simulink model "ADPSEMREMKNNash2015b"  (R2016a)
settings: Solver=ode1  StartTime=0.0  StopTime=40  FixedStep=1/1000  RelTol=1e-3  AbsTol=1e-3
PostLoadFcn:
  | f_Simulink_figureplace
InitFcn:
  | ADPSEMREMKNNash_PreSim
values from neighbouring files (symbols this model uses):
  beta1 = 0.3    [ADPSEMREMKNNash_PreSim.m]
  beta2 = 0.3    [ADPSEMREMKNNash_PreSim.m]
  beta3 = 0.3    [ADPSEMREMKNNash_PreSim.m]
  beta4 = 0.2    [ADPSEMREMKNNash_PreSim.m]
  beta5 = 0.1    [ADPSEMREMKNNash_PreSim.m]
  etaa11 = 1    [ADPSEMREMKNNash_PreSim.m]
  etaa12 = 0.5    [ADPSEMREMKNNash_PreSim.m]
  etaa13 = 1    [ADPSEMREMKNNash_PreSim.m]
  etaa14 = 0.5    [ADPSEMREMKNNash_PreSim.m]
  etaa15 = 1    [ADPSEMREMKNNash_PreSim.m]
  etaa21 = 2    [ADPSEMREMKNNash_PreSim.m]
  etaa22 = 1.5    [ADPSEMREMKNNash_PreSim.m]
  etaa23 = 2    [ADPSEMREMKNNash_PreSim.m]
  etaa24 = 1    [ADPSEMREMKNNash_PreSim.m]
  etaa25 = 1    [ADPSEMREMKNNash_PreSim.m]
  etac11 = 0.05    [ADPSEMREMKNNash_PreSim.m]
  etac12 = 0.001    [ADPSEMREMKNNash_PreSim.m]
  etac13 = 0.001    [ADPSEMREMKNNash_PreSim.m]
  etac14 = 0.001    [ADPSEMREMKNNash_PreSim.m]
  etac15 = 0.001    [ADPSEMREMKNNash_PreSim.m]
  etac21 = 5    [ADPSEMREMKNNash_PreSim.m]
  etac22 = 5    [ADPSEMREMKNNash_PreSim.m]
  etac23 = 5    [ADPSEMREMKNNash_PreSim.m]
  etac24 = 5    [ADPSEMREMKNNash_PreSim.m]
  etac25 = 5    [ADPSEMREMKNNash_PreSim.m]
  Gamma01 = 20*eye(L1)    [ADPSEMREMKNNash_PreSim.m]
  Gamma02 = 30*eye(L2)    [ADPSEMREMKNNash_PreSim.m]
  Gamma03 = 30*eye(L3)    [ADPSEMREMKNNash_PreSim.m]
  Gamma04 = 50*eye(L4)    [ADPSEMREMKNNash_PreSim.m]
  Gamma05 = 100*eye(L5)    [ADPSEMREMKNNash_PreSim.m]
  L5 = size(sig_p,1)    [ADPSEMREMKNN_Basis5.m]
  MovePoints = 1    [ADPSEMREMKNNash_PreSim.m]
  n = 3    [ADPSEMREMKNNash_PreSim.m]
  Q1 = [10 0 0; 0 10 0; 0 0 10]    [ADPSEMREMKNNash_PreSim.m]
  Q2 = [10 0 0; 0 10 0; 0 0 10]    [ADPSEMREMKNNash_PreSim.m]
  Q3 = [10 0 0; 0 10 0; 0 0 10]    [ADPSEMREMKNNash_PreSim.m]
  Q4 = [10 0 0; 0 10 0; 0 0 10]    [ADPSEMREMKNNash_PreSim.m]
  Q5 = [10 0 0; 0 10 0; 0 0 10]    [ADPSEMREMKNNash_PreSim.m]
  R1 = 1    [ADPSEMREMKNNash_PreSim.m]
  R2 = 1    [ADPSEMREMKNNash_PreSim.m]
  R3 = 1    [ADPSEMREMKNNash_PreSim.m]
  R4 = 1    [ADPSEMREMKNNash_PreSim.m]
  R5 = 1    [ADPSEMREMKNNash_PreSim.m]
  s1 = 0.25    [ADPSEMREMKNNash_PreSim.m]
  s2 = 0.25    [ADPSEMREMKNNash_PreSim.m]
  s3 = 0.25    [ADPSEMREMKNNash_PreSim.m]
  s4 = 0.25    [ADPSEMREMKNNash_PreSim.m]
  s5 = 0.25    [ADPSEMREMKNNash_PreSim.m]
  v1 = 1    [ADPSEMREMKNNash_PreSim.m]
  v2 = 1    [ADPSEMREMKNNash_PreSim.m]
  v3 = 1    [ADPSEMREMKNNash_PreSim.m]
  v4 = 1    [ADPSEMREMKNNash_PreSim.m]
  v5 = 1    [ADPSEMREMKNNash_PreSim.m]
  WaH01 = 2*ones(L1,1)    [ADPSEMREMKNNash_PreSim.m]
  WaH02 = 2*ones(L2,1)    [ADPSEMREMKNNash_PreSim.m]
  WaH03 = 2*ones(L3,1)    [ADPSEMREMKNNash_PreSim.m]
  WaH04 = 1*ones(L4,1)    [ADPSEMREMKNNash_PreSim.m]
  WaH05 = 1*ones(L5,1)    [ADPSEMREMKNNash_PreSim.m]
  WcH01 = 5*ones(L1,1)    [ADPSEMREMKNNash_PreSim.m]
  WcH02 = 2*ones(L2,1)    [ADPSEMREMKNNash_PreSim.m]
  WcH03 = 2*ones(L3,1)    [ADPSEMREMKNNash_PreSim.m]
  WcH04 = 5*ones(L4,1)    [ADPSEMREMKNNash_PreSim.m]
  WcH05 = 2*ones(L5,1)    [ADPSEMREMKNNash_PreSim.m]
  x01 = [0; 0; 0]    [ADPSEMREMKNNash_PreSim.m]
  x02 = [0; 0; 0]    [ADPSEMREMKNNash_PreSim.m]
  x03 = [0; 0; 0]    [ADPSEMREMKNNash_PreSim.m]
  x04 = 0*[0.5; -0.5; 0]    [ADPSEMREMKNNash_PreSim.m]
  x05 = 0*[-0.5; -0.5; 0]    [ADPSEMREMKNNash_PreSim.m]
  xd21 = [0.5;-0.5;0]    [ADPSEMREMKNN_Plot.m]    (also in ADPSEMREMKNNash_PreSim.m)
  xd23 = xd21-xd31    [ADPSEMREMKNN_Plot.m]    (also in ADPSEMREMKNNash_PreSim.m)
  xd31 = [-0.5;-0.5;0]    [ADPSEMREMKNN_Plot.m]    (also in ADPSEMREMKNNash_PreSim.m)
  xd40 = [0.5;0.5;0]    [ADPSEMREMKNN_Plot.m]    (also in ADPSEMREMKNNash_PreSim.m)
  xd45 = [1;0;0]    [ADPSEMREMKNNash_PreSim.m]
  xd54 = [-1;0;0]    [ADPSEMREMKNNash_PreSim.m]
settings Model: Creator=rkamalapurkar  LastModifiedBy=rlkam
settings DataIOCC: SaveFormat=Array  SaveOutput=off  DSMLogging=off  SaveTime=off  SignalLoggingName=ADPSEMREMKNNData
settings OptimizationCC: ExpressionDepthLimit=2147483647  SimCompilerOptimization=on
settings DebuggingCC: UnderspecifiedInitializationDetection=Classic  MergeDetectMultiDrivingBlocksExec=none  SolverPrmCheckMsg=warning  FcnCallInpInsideContextMsg=UseLocalSettings  StateNameClashWarn=warning
settings HardwareCC: ProdBitPerPointer=32  ProdLargestAtomicFloat=None  ProdIntDivRoundTo=Undefined  ProdEndianess=Unspecified  ProdWordSize=32  ProdHWDeviceType=32-bit Generic
settings ModelReferenceCC: PropagateSignalLabelsOutOfModel=off
settings GRTTargetCC: CombineOutputUpdateFcns=off  GRTInterface=on
settings ConfigComp: CovModelRefEnable=Off  CovSFcnEnable=off

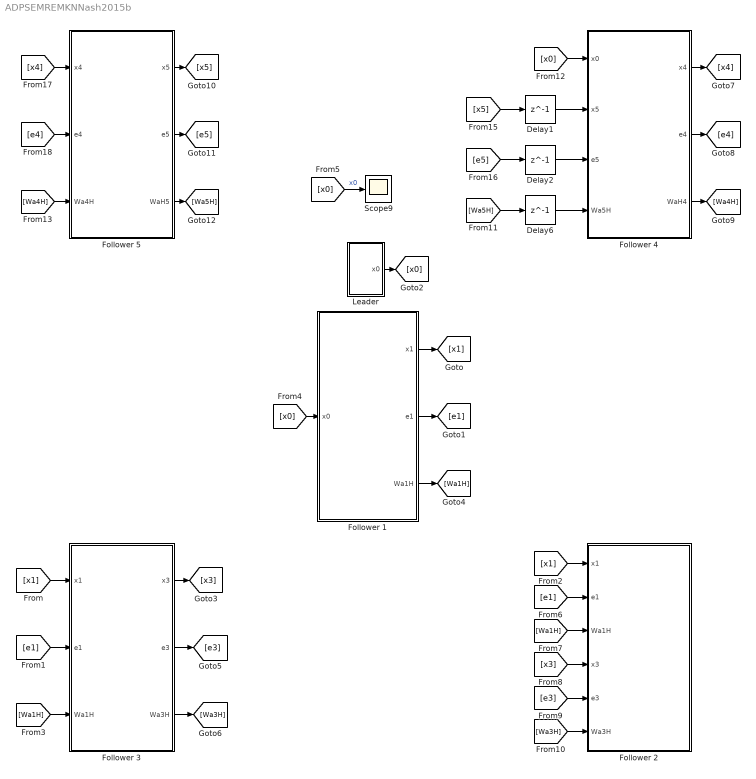
== system ADPSEMREMKNNash2015b ==
  Delay1 : Delay  DelayLength=1  InitialCondition=x05
  Delay2 : Delay  DelayLength=1  InitialCondition=zeros(3,1)
  Delay6 : Delay  DelayLength=1  InitialCondition=zeros(L5,1)
  Follower 1 : Subsystem
  Follower 2 : Subsystem
  Follower 3 : Subsystem
  Follower 4 : Subsystem
  Follower 5 : Subsystem
  Leader : Subsystem
  Scope9 : Scope
  wires:
  Leader/1(x0) -> [x0]
  [x0] -> Follower 1/1(x0)
  [x0] -> Scope9/1  "x0"
  Follower 1/1(x1) -> [x1]
  Follower 1/2(e1) -> [e1]
  Follower 1/3(Wa1H) -> [Wa1H]
  [x1] -> Follower 3/1(x1)
  [e1] -> Follower 3/2(e1)
  [Wa1H] -> Follower 3/3(Wa1H)
  Follower 3/1(x3) -> [x3]
  Follower 3/2(e3) -> [e3]
  Follower 3/3(Wa3H) -> [Wa3H]
  [x1] -> Follower 2/1(x1)
  [e1] -> Follower 2/2(e1)
  [Wa1H] -> Follower 2/3(Wa1H)
  [x3] -> Follower 2/4(x3)
  [e3] -> Follower 2/5(e3)
  [Wa3H] -> Follower 2/6(Wa3H)
  [x0] -> Follower 4/1(x0)
  [x4] -> Follower 5/1(x4)
  [Wa4H] -> Follower 5/3(Wa4H)
  Follower 4/1(x4) -> [x4]
  Follower 4/2(e4) -> [e4]
  Follower 4/3(WaH4) -> [Wa4H]
  Follower 5/1(x5) -> [x5]
  Follower 5/2(e5) -> [e5]
  Follower 5/3(WaH5) -> [Wa5H]
  [e4] -> Follower 5/2(e4)
  [e5] -> Delay2/1
  [Wa5H] -> Delay6/1
  [x5] -> Delay1/1
  Delay1/1 -> Follower 4/2(x5)
  Delay2/1 -> Follower 4/3(e5)
  Delay6/1 -> Follower 4/4(Wa5H)

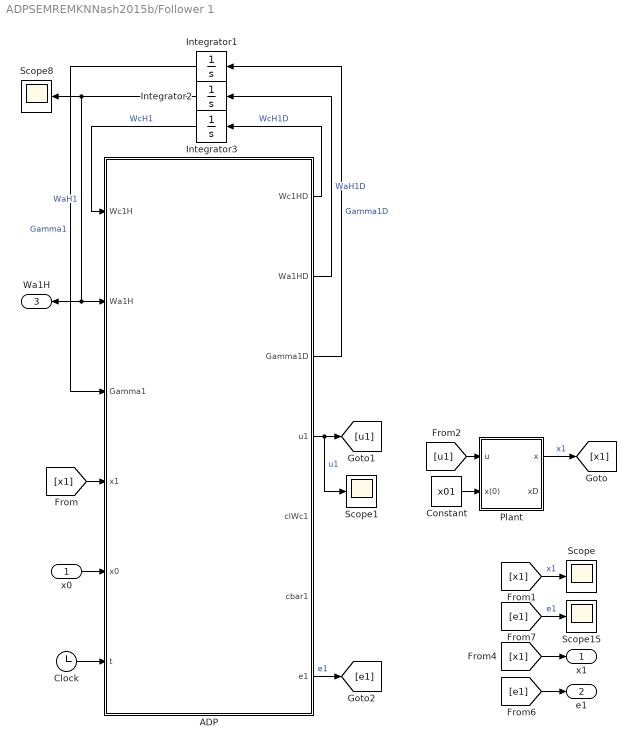
== system ADPSEMREMKNNash2015b/Follower 1 ==
  x0 : Inport
  ADP : MATLAB Function  TreatAsAtomicUnit=on
  Clock : Clock
  Constant : Constant  Value=x01
  Integrator1 : Integrator  InitialCondition=Gamma01
  Integrator2 : Integrator  InitialCondition=WaH01
  Integrator3 : Integrator  InitialCondition=WcH01
  Plant : Subsystem
  Scope{,1,8,15} (4 alike) : Scope
  x1 : Outport
  e1 : Outport  Port=2
  Wa1H : Outport  Port=3
  wires:
  Integrator2/1 -> ADP/2(Wa1H), Wa1H/1, Scope8/1  "WaH1"
  ADP/3(Gamma1D) -> Integrator1/1  "Gamma1D"
  Integrator3/1 -> ADP/1(Wc1H)  "WcH1"
  Plant/1(x) -> [x1]  "x1"
  Constant/1 -> Plant/2(x(0))
  ADP/1(Wc1HD) -> Integrator3/1  "WcH1D"
  Clock/1 -> ADP/6(t)
  [x1] -> ADP/4(x1)
  ADP/2(Wa1HD) -> Integrator2/1  "WaH1D"
  x0/1 -> ADP/5(x0)
  [u1] -> Plant/1(u)
  [x1] -> Scope/1  "x1"
  ADP/4(u1) -> Scope1/1, [u1]  "u1"
  Integrator1/1 -> ADP/3(Gamma1)  "Gamma1"
  [x1] -> x1/1
  ADP/7(e1) -> [e1]  "e1"
  [e1] -> e1/1
  [e1] -> Scope15/1  "e1"

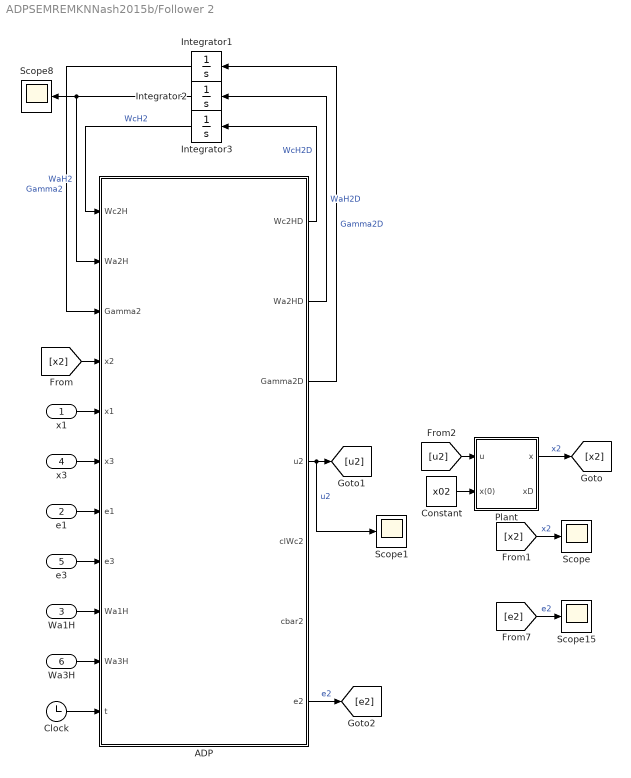
== system ADPSEMREMKNNash2015b/Follower 2 ==
  x1 : Inport
  e1 : Inport  Port=2
  Wa1H : Inport  Port=3
  x3 : Inport  Port=4
  e3 : Inport  Port=5
  Wa3H : Inport  Port=6
  ADP : MATLAB Function  TreatAsAtomicUnit=on
  Clock : Clock
  Constant : Constant  Value=x02
  Integrator1 : Integrator  InitialCondition=Gamma02
  Integrator2 : Integrator  InitialCondition=WaH02
  Integrator3 : Integrator  InitialCondition=WcH02
  Plant : Subsystem
  Scope{,1,8,15} (4 alike) : Scope
  wires:
  Integrator2/1 -> ADP/2(Wa2H), Scope8/1  "WaH2"
  ADP/3(Gamma2D) -> Integrator1/1  "Gamma2D"
  Integrator3/1 -> ADP/1(Wc2H)  "WcH2"
  Plant/1(x) -> [x2]  "x2"
  Constant/1 -> Plant/2(x(0))
  ADP/1(Wc2HD) -> Integrator3/1  "WcH2D"
  Clock/1 -> ADP/11(t)
  ADP/2(Wa2HD) -> Integrator2/1  "WaH2D"
  x1/1 -> ADP/5(x1)
  [u2] -> Plant/1(u)
  [x2] -> Scope/1  "x2"
  ADP/4(u2) -> Scope1/1, [u2]  "u2"
  Integrator1/1 -> ADP/3(Gamma2)  "Gamma2"
  ADP/7(e2) -> [e2]  "e2"
  [e2] -> Scope15/1  "e2"
  e1/1 -> ADP/7(e1)
  Wa1H/1 -> ADP/9(Wa1H)
  [x2] -> ADP/4(x2)
  x3/1 -> ADP/6(x3)
  e3/1 -> ADP/8(e3)
  Wa3H/1 -> ADP/10(Wa3H)

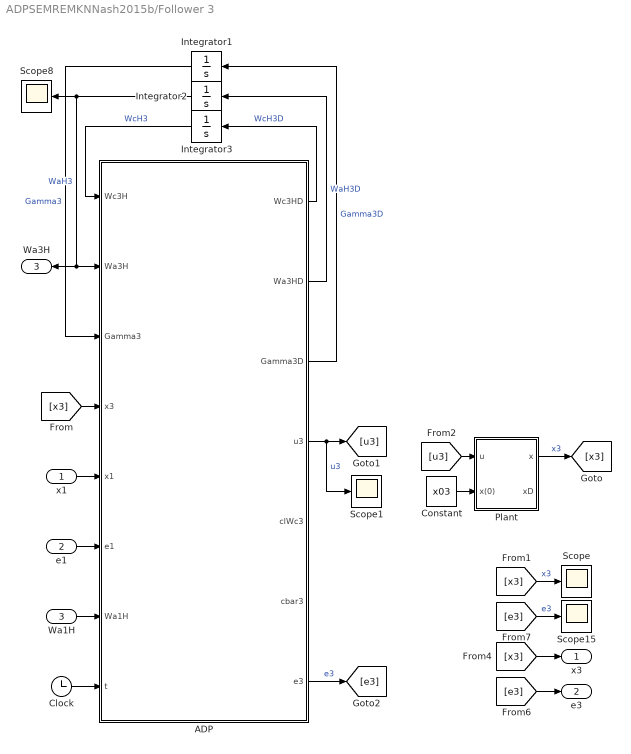
== system ADPSEMREMKNNash2015b/Follower 3 ==
  x1 : Inport
  e1 : Inport  Port=2
  Wa1H : Inport  Port=3
  ADP : MATLAB Function  TreatAsAtomicUnit=on
  Clock : Clock
  Constant : Constant  Value=x03
  Integrator1 : Integrator  InitialCondition=Gamma03
  Integrator2 : Integrator  InitialCondition=WaH03
  Integrator3 : Integrator  InitialCondition=WcH03
  Plant : Subsystem
  Scope{,1,8,15} (4 alike) : Scope
  x3 : Outport
  e3 : Outport  Port=2
  Wa3H : Outport  Port=3
  wires:
  Integrator2/1 -> Scope8/1, ADP/2(Wa3H), Wa3H/1  "WaH3"
  ADP/3(Gamma3D) -> Integrator1/1  "Gamma3D"
  Integrator3/1 -> ADP/1(Wc3H)  "WcH3"
  Plant/1(x) -> [x3]  "x3"
  Constant/1 -> Plant/2(x(0))
  ADP/1(Wc3HD) -> Integrator3/1  "WcH3D"
  Clock/1 -> ADP/8(t)
  [x3] -> ADP/4(x3)
  ADP/2(Wa3HD) -> Integrator2/1  "WaH3D"
  x1/1 -> ADP/5(x1)
  [u3] -> Plant/1(u)
  [x3] -> Scope/1  "x3"
  ADP/4(u3) -> Scope1/1, [u3]  "u3"
  Integrator1/1 -> ADP/3(Gamma3)  "Gamma3"
  [x3] -> x3/1
  ADP/7(e3) -> [e3]  "e3"
  [e3] -> e3/1
  [e3] -> Scope15/1  "e3"
  e1/1 -> ADP/6(e1)
  Wa1H/1 -> ADP/7(Wa1H)

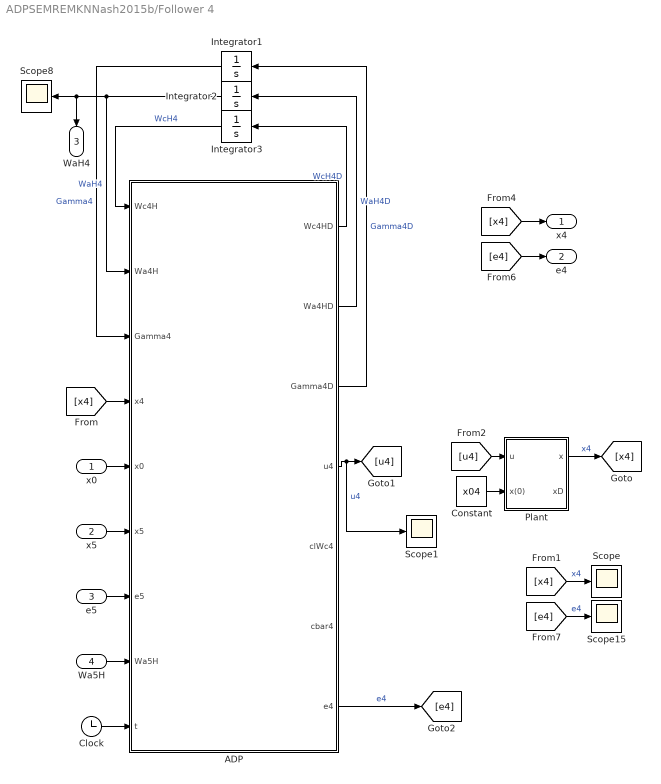
== system ADPSEMREMKNNash2015b/Follower 4 ==
  x0 : Inport
  x5 : Inport  Port=2
  e5 : Inport  Port=3
  Wa5H : Inport  Port=4
  ADP : MATLAB Function  TreatAsAtomicUnit=on
  Clock : Clock
  Constant : Constant  Value=x04
  Integrator1 : Integrator  InitialCondition=Gamma04
  Integrator2 : Integrator  InitialCondition=WaH04
  Integrator3 : Integrator  InitialCondition=WcH04
  Plant : Subsystem
  Scope{,1,8,15} (4 alike) : Scope
  x4 : Outport
  e4 : Outport  Port=2
  WaH4 : Outport  Port=3
  wires:
  Integrator2/1 -> ADP/2(Wa4H), WaH4/1, Scope8/1  "WaH4"
  ADP/3(Gamma4D) -> Integrator1/1  "Gamma4D"
  Integrator3/1 -> ADP/1(Wc4H)  "WcH4"
  Plant/1(x) -> [x4]  "x4"
  Constant/1 -> Plant/2(x(0))
  ADP/1(Wc4HD) -> Integrator3/1  "WcH4D"
  Clock/1 -> ADP/9(t)
  ADP/2(Wa4HD) -> Integrator2/1  "WaH4D"
  x0/1 -> ADP/5(x0)
  [u4] -> Plant/1(u)
  [x4] -> Scope/1  "x4"
  ADP/4(u4) -> Scope1/1, [u4]  "u4"
  Integrator1/1 -> ADP/3(Gamma4)  "Gamma4"
  ADP/7(e4) -> [e4]  "e4"
  [e4] -> Scope15/1  "e4"
  [x4] -> ADP/4(x4)
  x5/1 -> ADP/6(x5)
  e5/1 -> ADP/7(e5)
  Wa5H/1 -> ADP/8(Wa5H)
  [e4] -> e4/1
  [x4] -> x4/1

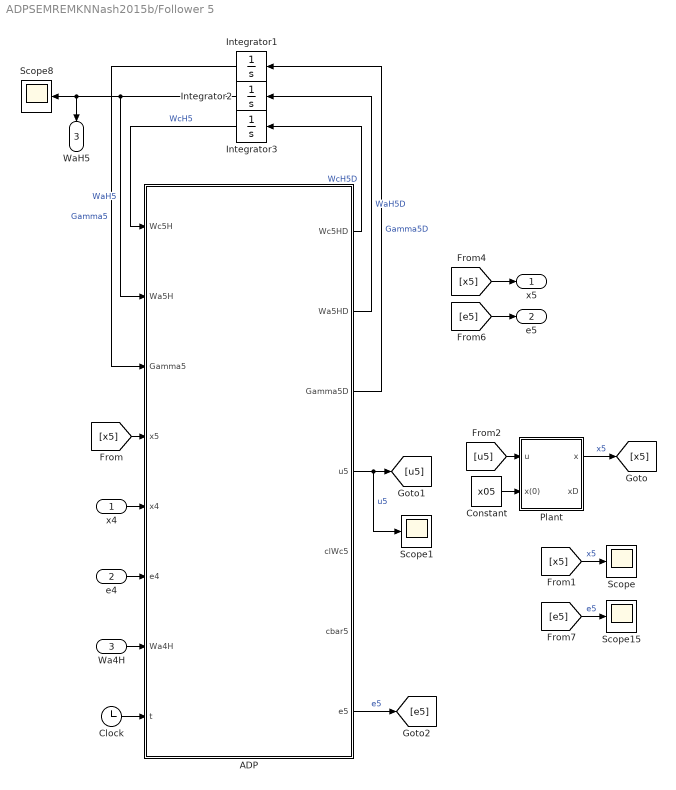
== system ADPSEMREMKNNash2015b/Follower 5 ==
  x4 : Inport
  e4 : Inport  Port=2
  Wa4H : Inport  Port=3
  ADP : MATLAB Function  TreatAsAtomicUnit=on
  Clock : Clock
  Constant : Constant  Value=x05
  Integrator1 : Integrator  InitialCondition=Gamma05
  Integrator2 : Integrator  InitialCondition=WaH05
  Integrator3 : Integrator  InitialCondition=WcH05
  Plant : Subsystem
  Scope{,1,8,15} (4 alike) : Scope
  x5 : Outport
  e5 : Outport  Port=2
  WaH5 : Outport  Port=3
  wires:
  Integrator2/1 -> ADP/2(Wa5H), WaH5/1, Scope8/1  "WaH5"
  ADP/3(Gamma5D) -> Integrator1/1  "Gamma5D"
  Integrator3/1 -> ADP/1(Wc5H)  "WcH5"
  Plant/1(x) -> [x5]  "x5"
  Constant/1 -> Plant/2(x(0))
  ADP/1(Wc5HD) -> Integrator3/1  "WcH5D"
  Clock/1 -> ADP/8(t)
  ADP/2(Wa5HD) -> Integrator2/1  "WaH5D"
  [u5] -> Plant/1(u)
  [x5] -> Scope/1  "x5"
  ADP/4(u5) -> Scope1/1, [u5]  "u5"
  Integrator1/1 -> ADP/3(Gamma5)  "Gamma5"
  ADP/7(e5) -> [e5]  "e5"
  [e5] -> Scope15/1  "e5"
  e4/1 -> ADP/6(e4)
  Wa4H/1 -> ADP/7(Wa4H)
  [x5] -> ADP/4(x5)
  x4/1 -> ADP/5(x4)
  [e5] -> e5/1
  [x5] -> x5/1

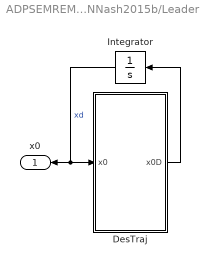
== system ADPSEMREMKNNash2015b/Leader ==
  DesTraj : MATLAB Function  TreatAsAtomicUnit=on
  Integrator : Integrator  InitialCondition=[0;-1;0]
  x0 : Outport
  wires:
  DesTraj/1(x0D) -> Integrator/1
  Integrator/1 -> x0/1, DesTraj/1(x0)  "xd"

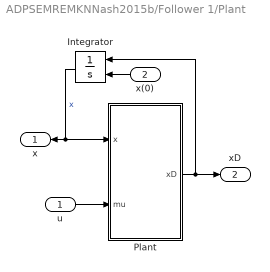
== system ADPSEMREMKNNash2015b/Follower 1/Plant ==
  u : Inport
  x(0) : Inport  Port=2
  Integrator : Integrator  InitialConditionSource=external  InitialCondition=[1;1;0.0;0.0]
  Plant : MATLAB Function  TreatAsAtomicUnit=on
  x : Outport
  xD : Outport  Port=2
  wires:
  Plant/1(xD) -> Integrator/1, xD/1
  Integrator/1 -> Plant/1(x), x/1  "x"
  u/1 -> Plant/2(mu)
  x(0)/1 -> Integrator/2

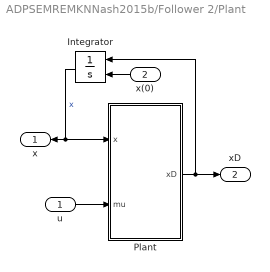
== system ADPSEMREMKNNash2015b/Follower 2/Plant ==
  u : Inport
  x(0) : Inport  Port=2
  Integrator : Integrator  InitialConditionSource=external  InitialCondition=[1;1;0.0;0.0]
  Plant : MATLAB Function  TreatAsAtomicUnit=on
  x : Outport
  xD : Outport  Port=2
  wires:
  Plant/1(xD) -> Integrator/1, xD/1
  Integrator/1 -> Plant/1(x), x/1  "x"
  u/1 -> Plant/2(mu)
  x(0)/1 -> Integrator/2

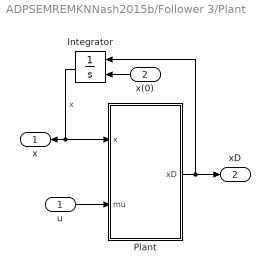
== system ADPSEMREMKNNash2015b/Follower 3/Plant ==
  u : Inport
  x(0) : Inport  Port=2
  Integrator : Integrator  InitialConditionSource=external  InitialCondition=[1;1;0.0;0.0]
  Plant : MATLAB Function  TreatAsAtomicUnit=on
  x : Outport
  xD : Outport  Port=2
  wires:
  Plant/1(xD) -> Integrator/1, xD/1
  Integrator/1 -> Plant/1(x), x/1  "x"
  u/1 -> Plant/2(mu)
  x(0)/1 -> Integrator/2

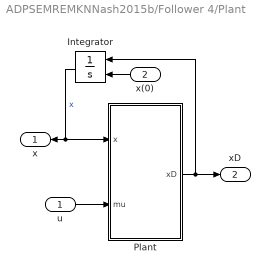
== system ADPSEMREMKNNash2015b/Follower 4/Plant ==
  u : Inport
  x(0) : Inport  Port=2
  Integrator : Integrator  InitialConditionSource=external  InitialCondition=[1;1;0.0;0.0]
  Plant : MATLAB Function  TreatAsAtomicUnit=on
  x : Outport
  xD : Outport  Port=2
  wires:
  Plant/1(xD) -> Integrator/1, xD/1
  Integrator/1 -> Plant/1(x), x/1  "x"
  u/1 -> Plant/2(mu)
  x(0)/1 -> Integrator/2

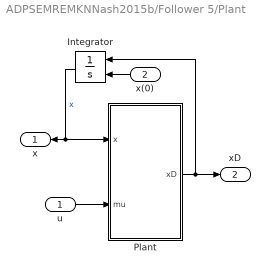
== system ADPSEMREMKNNash2015b/Follower 5/Plant ==
  u : Inport
  x(0) : Inport  Port=2
  Integrator : Integrator  InitialConditionSource=external  InitialCondition=[1;1;0.0;0.0]
  Plant : MATLAB Function  TreatAsAtomicUnit=on
  x : Outport
  xD : Outport  Port=2
  wires:
  Plant/1(xD) -> Integrator/1, xD/1
  Integrator/1 -> Plant/1(x), x/1  "x"
  u/1 -> Plant/2(mu)
  x(0)/1 -> Integrator/2

== matlab function ADPSEMREMKNNash2015b/Leader/DesTraj ==
  data: x0D output; x0 input
function x0D = DesTraj(x0)
%#codegen
[ x0D, ~ ] = gen0( x0 );








% % xd1(t)=cos(t);
% % xd2(t)=sin(t)*cos(t);
% % xd3(t)=sin(t);
% xdD = [-xd(3);xd(1)^2-xd(3)^2;xd(1)];
% 
% % G=[1 0;0 1;-x(2) x(1)];
% % 
% % % gplus=
% % (1/(x1^2 + x2^2 + 1))*[...
% % [ (x1^2 + 1),    (x1*x2), -x2]
% % [    (x1*x2), (x2^2 + 1),  x1]];

== matlab function ADPSEMREMKNNash2015b/Follower 1/ADP ==
  data: Wc1H input; Wa1H input; Gamma1 input; x1 input; x0 input; t input; R1 parameter; Q1 parameter; etaa11 parameter; etaa21 parameter; etac11 parameter; v1 parameter; Wc1HD output; Wa1HD output; Gamma1D output; u1 output; clWc1 output; cbar1 output; etac21 parameter; beta1 parameter; n parameter; e1 output; s1 parameter; MovePoints parameter; xd31 parameter; xd21 parameter; xd23 parameter
function [Wc1HD,Wa1HD,Gamma1D,u1,clWc1,cbar1,e1]=...
    control(Wc1H,Wa1H,Gamma1,x1,x0,t,R1,Q1,etaa11,etaa21,etac11,v1,...
    etac21,beta1,n,s1,MovePoints,xd31, xd21, xd23)
%#codegen
e1 = x1-x0;
% Z = [e1;x0];
calE1=[e1;x1];

%% ADP
[ mu1,scrG1,scrF1,calG1,calF1,Gsig1 ] = gen1( calE1,Wa1H,R1 );
[~,sig1GRe1,sig1GRx1,~]=ADPSEMREMKNN_Basis1(calE1);   
omega1 = sig1GRe1*(scrF1+scrG1*mu1)+sig1GRx1*(calF1+calG1*mu1);
r = e1'*Q1*e1 + mu1'*R1*mu1;
delta1 = Wc1H'*omega1 + r;
rho = (1+v1*(omega1'*omega1));
[ ~, f10 ] = gen0( x0 );
u10 = f10;
%% Concurrent Learning
TimePeriod = 6*pi;
FreqParam = 0.1;
if MovePoints == 0
    temp=linspace(-s1,s1,3);
    ttemp=linspace(0,TimePeriod,10);
    [temp1, temp2, temp3, temp4] = ndgrid(temp,temp,temp,ttemp);
    EC=[temp1(:) temp2(:) temp3(:)]'; % matrix with columns as selected points
    TC=temp4(:)';
    X0C=[sin(TimePeriod*tanh(FreqParam*TC)); ...
        -cos(TimePeriod*tanh(FreqParam*TC)); TimePeriod*tanh(FreqParam*TC)];
    xd31=[-0.5;-0.5;0];
    xd21=[0.5;-0.5;0];
    xd23=xd21-xd31;
    XC=[EC(1:3,:)+X0C;...
        (1/2)*(2*EC(1:3,:)+EC(4:6,:)+EC(7:9,:)+xd21+xd31+xd23+2*X0C);...
        EC(1:3,:)+EC(7:9,:)+xd31+X0C;...
        ];
    N = size(XC,2); %Number of points
else
    N=1;
    NN=1;
    EC=unifrnd(-s1,s1,3*n,N);
    TC=unifrnd(0,1*TimePeriod,1,NN);
    X0C=[sin(TimePeriod*tanh(FreqParam*TC)); ...
    -cos(TimePeriod*tanh(FreqParam*TC)); TimePeriod*tanh(FreqParam*TC)];
    XC=[EC(1:3,:)+X0C;...
        (1/2)*(2*EC(1:3,:)+EC(4:6,:)+EC(7:9,:)+xd21+xd31+xd23+2*X0C);...
        EC(1:3,:)+EC(7:9,:)+xd31+X0C;...
        ];
end
clWc1=zeros(size(Wc1H));
clWa1=zeros(size(Wa1H));
CLmatrix1=zeros(size(Wc1H,1),size(Wc1H,1));
CLGamma1=zeros(size(Gamma1));
parfor i=1:N
    e1i=EC(1:n,i);
    x1i=XC(1:n,i);
    calE1i=[e1i;x1i];
    [ mu1i,scrG1i,scrF1i,calG1i,calF1i,Gsig1i ] = gen1( calE1i,Wa1H,R1 );
    [~,sig1GRe1i,sig1GRx1i,~]=ADPSEMREMKNN_Basis1(calE1i);   
    omega1i = sig1GRe1i*(scrF1i+scrG1i*mu1i)+sig1GRx1i*(calF1i+calG1i*mu1i);
    ri = e1i'*Q1*e1i + mu1i'*R1*mu1i;
    delta1i = Wc1H'*omega1i + ri;
    rho1i = (1+v1*(omega1i'*omega1i));
    clWc1=clWc1+Gamma1*omega1i*delta1i/rho1i;
    clWa1=clWa1+(Gsig1i'*(R1\Gsig1i))*Wa1H*omega1i'*Wc1H/(4*rho1i);
    CLmatrix1=CLmatrix1+omega1i*omega1i'/(N*rho1i);
    CLGamma1=CLGamma1+Gamma1*(omega1i*omega1i'/rho1i^2)*Gamma1;
end
clWc1=-etac21*clWc1/N;
clWa1=etac21*clWa1/N;
CLGamma1=CLGamma1/N;
cbar1=real(min(svd(CLmatrix1)));

%% Update Laws

Wc1HD = (-etac11*Gamma1*omega1*delta1/rho+clWc1);
Gamma1D = (beta1*Gamma1-Gamma1*(omega1*omega1'/rho^2)*Gamma1-CLGamma1);
Wa1HD = etaa11*(Wc1H-Wa1H)-etaa21*Wa1H...
    -(-etac11*(Gsig1'*(R1\Gsig1))*Wa1H*omega1'*Wc1H/(4*rho))+clWa1;
%% Controller
u1 = mu1+u10;
% u1 = -100*g1'*e1+u10;

== matlab function ADPSEMREMKNNash2015b/Follower 1/Plant/Plant ==
  data: xD output; x input; mu input
function xD = dynamics(x,mu)
%#codegen
F=0;
G=[cos(x(3)) 0;sin(x(3)) 0;0 1];
xD = F+G*mu;

% G=[1 0;0 1;-x(2) x(1)];
% 
% % gplus=
% (1/(x1^2 + x2^2 + 1))*[...
% [ (x1^2 + 1),    (x1*x2), -x2]
% [    (x1*x2), (x2^2 + 1),  x1]];

== matlab function ADPSEMREMKNNash2015b/Follower 3/ADP ==
  data: Wc3H input; Wa3H input; Gamma3 input; x3 input; x1 input; e1 input; Wa1H input; t input; R3 parameter; R1 parameter; Q3 parameter; etaa13 parameter; etaa23 parameter; etac13 parameter; v3 parameter; Wc3HD output; Wa3HD output; Gamma3D output; u3 output; clWc3 output; cbar3 output; etac23 parameter; beta3 parameter; n parameter; e3 output; s3 parameter; MovePoints parameter; xd31 parameter; xd21 parameter; xd23 parameter
function [Wc3HD,Wa3HD,Gamma3D,u3,clWc3,cbar3,e3]=...
    control(Wc3H,Wa3H,Gamma3,x3,x1,e1,Wa1H,t,R3,R1,Q3,etaa13,etaa23,etac13,v3,...
    etac23,beta3,n,s3,MovePoints,xd31, xd21, xd23)
%#codegen
e3 = x3-x1-xd31;
% Z = [e1;x0];
calE3=[e3;e1;x3];
calE1=[e1;x1];
%% ADP
[ mu1,scrG1,scrF1,~,~,~ ] = gen1( calE1,Wa1H,R1 );
[ mu3,scrG3,scrF3,calG3,calF3,Gsig3,F3 ] = gen3( calE3,calE1,Wa3H,R3 );
[~,sig3GRe3,sig3GRx3,sig3GRe1,~]=ADPSEMREMKNN_Basis3(calE3); 
muS3=[mu3;mu1];
muS1=mu1;
omega3 = sig3GRe3*(scrF3+scrG3*muS3)+sig3GRx3*(calF3+calG3*muS3)+sig3GRe1*(scrF1+scrG1*muS1);
r = e3'*Q3*e3 + mu3'*R3*mu3;
delta1 = Wc3H'*omega3 + r;
rho3 = (1+v3*(omega3'*omega3));
scrLg33=[eye(2) eye(2)];
%% Concurrent Learning
TimePeriod = 6*pi;
FreqParam = 0.1;
if MovePoints == 0
    temp=linspace(-s3,s3,3);
    ttemp=linspace(0,TimePeriod,10);
    [temp1, temp2, temp3, temp4] = ndgrid(temp,temp,temp,ttemp);
    EC=[temp1(:) temp2(:) temp3(:)]'; % matrix with columns as selected points
    TC=temp4(:)';
    X0C=[sin(TimePeriod*tanh(FreqParam*TC)); ...
        -cos(TimePeriod*tanh(FreqParam*TC)); TimePeriod*tanh(FreqParam*TC)];
    xd31=[-0.5;-0.5;0];
    xd21=[0.5;-0.5;0];
    xd23=xd21-xd31;
    XC=[EC(1:3,:)+X0C;...
        (1/2)*(2*EC(1:3,:)+EC(4:6,:)+EC(7:9,:)+xd21+xd31+xd23+2*X0C);...
        EC(1:3,:)+EC(7:9,:)+xd31+X0C;...
        ];
    N = size(XC,2); %Number of points
else
    N=1;
    NN=1;
    EC=unifrnd(-s3,s3,3*n,N);
    TC=unifrnd(0,1*TimePeriod,1,NN);
    X0C=[sin(TimePeriod*tanh(FreqParam*TC)); ...
    -cos(TimePeriod*tanh(FreqParam*TC)); TimePeriod*tanh(FreqParam*TC)];
    XC=[EC(1:3,:)+X0C;...
        (1/2)*(2*EC(1:3,:)+EC(4:6,:)+EC(7:9,:)+xd21+xd31+xd23+2*X0C);...
        EC(1:3,:)+EC(7:9,:)+xd31+X0C;...
        ];
end
clWc3=zeros(size(Wc3H));
clWa3=zeros(size(Wa3H));
CLmatrix3=zeros(size(Wc3H,1),size(Wc3H,1));
CLGamma3=zeros(size(Gamma3));
parfor i=1:N
    e1i=EC(1:n,i);
    x1i=XC(1:n,i);
    e3i=EC(7:9,i);
    x3i=XC(7:9,i);
    calE1i=[e1i;x1i];
    calE3i=[e3i;e1i;x3i];
    [ mu1i,scrG1i,scrF1i,~,~,~ ] = gen1( calE1i,Wa1H,R1 );
    [ mu3i,scrG3i,scrF3i,calG3i,calF3i,Gsig3i,~ ] = gen3( calE3i,calE1i,Wa3H,R3 );
    [~,sig3GRe3i,sig3GRx3i,sig3GRe1i,~]=ADPSEMREMKNN_Basis3(calE3i);
    muS3i=[mu3i;mu1i];
    muS1i=mu1i;
    omega3i = sig3GRe3i*(scrF3i+scrG3i*muS3i)+sig3GRx3i*(calF3i+calG3i*muS3i)+sig3GRe1i*(scrF1i+scrG1i*muS1i);
    ri = e3i'*Q3*e3i + mu3i'*R3*mu3i;
    delta3i = Wc3H'*omega3i + ri;
    rho3i = (1+v3*(omega3i'*omega3i));
    clWc3=clWc3+Gamma3*omega3i*delta3i/rho3i;
    clWa3=clWa3+(Gsig3i'*(R3\Gsig3i))*Wa3H*omega3i'*Wc3H/(4*rho3i);
    CLmatrix3=CLmatrix3+omega3i*omega3i'/(N*rho3i);
    CLGamma3=CLGamma3+Gamma3*(omega3i*omega3i'/rho3i^2)*Gamma3;
end
clWc3=-etac23*clWc3/N;
clWa3=etac23*clWa3/N;
CLGamma3=CLGamma3/N;
cbar3=real(min(svd(CLmatrix3)));

%% Update Laws

Wc3HD = (-etac13*Gamma3*omega3*delta1/rho3+clWc3);
Gamma3D = (beta3*Gamma3-Gamma3*(omega3*omega3'/rho3^2)*Gamma3-CLGamma3);
Wa3HD = etaa13*(Wc3H-Wa3H)...
    -(etaa23*Wa3H-etac13*(Gsig3'*(R3\Gsig3))*Wa3H*omega3'*Wc3H/(4*rho3))+clWa3;
%% Controller
u3 = scrLg33*(muS3+F3);
% u1 = -100*g1'*e1+u10;

== matlab function ADPSEMREMKNNash2015b/Follower 3/Plant/Plant ==
  data: xD output; x input; mu input
function xD = dynamics(x,mu)
%#codegen
F=0;
G=[cos(x(3)) 0;sin(x(3)) 0;0 1];
xD = F+G*mu;

% G=[1 0;0 1;-x(2) x(1)];
% 
% % gplus=
% (1/(x1^2 + x2^2 + 1))*[...
% [ (x1^2 + 1),    (x1*x2), -x2]
% [    (x1*x2), (x2^2 + 1),  x1]];

== matlab function ADPSEMREMKNNash2015b/Follower 2/ADP ==
  data: Wc2H input; Wa2H input; Gamma2 input; x2 input; x1 input; x3 input; e1 input; e3 input; Wa1H input; Wa3H input; t input; R2 parameter; R1 parameter; R3 parameter; Q2 parameter; etaa12 parameter; Wc2HD output; Wa2HD output; Gamma2D output; u2 output; clWc2 output; cbar2 output; etaa22 parameter; etac12 parameter; v2 parameter; etac22 parameter; beta2 parameter; n parameter; s2 parameter; MovePoints parameter; xd31 parameter; xd21 parameter; xd23 parameter; e2 output
function [Wc2HD,Wa2HD,Gamma2D,u2,clWc2,cbar2,e2]=...
    control(Wc2H,Wa2H,Gamma2,x2,x1,x3,e1,e3,Wa1H,Wa3H,t,R2,R1,R3,Q2,etaa12,etaa22,etac12,v2,...
    etac22,beta2,n,s2,MovePoints,xd31,xd21,xd23)
%#codegen
e2 = x2-x1-xd21+x2-x3-xd23;
% Z = [e1;x0];
calE2=[e2;e1;e3;x2];
calE1=[e1;x1];
calE3=[e2;e1;x2];
%% ADP
[ mu1,scrG1,scrF1,~,~,~ ] = gen1( calE1,Wa1H,R1 );
[ mu3,scrG3,scrF3,~,~,~,~ ] = gen3( calE3,calE1,Wa3H,R3 );
[ mu2,scrG2,scrF2,calG2,calF2,Gsig2,F2 ] = gen2( calE2,calE1,calE3,Wa2H,R2 );
[~,sig2GRe2,sig2GRx2,sig2GRe1,sig2GRe3,~]=ADPSEMREMKNN_Basis2(calE2); 
muS2=[mu2;mu1;mu3];
muS3=[mu3;mu1];
muS1=mu1;
omega2 = sig2GRe2*(scrF2+scrG2*muS2)+sig2GRx2*(calF2+calG2*muS2)...
    +sig2GRe1*(scrF1+scrG1*muS1)+sig2GRe3*(scrF3+scrG3*muS3);
r = e2'*Q2*e2 + mu2'*R2*mu2;
delta2 = Wc2H'*omega2 + r;
rho2 = (1+v2*(omega2'*omega2));
scrLg22=[0.5*eye(2) eye(2) 0.5*eye(2)];
%% Concurrent Learning
TimePeriod = 6*pi;
FreqParam = 0.1;
if MovePoints == 0
    temp=linspace(-s2,s2,3);
    ttemp=linspace(0,TimePeriod,10);
    [temp1, temp2, temp3, temp4] = ndgrid(temp,temp,temp,ttemp);
    EC=[temp1(:) temp2(:) temp3(:)]'; % matrix with columns as selected points
    TC=temp4(:)';
    X0C=[sin(TimePeriod*tanh(FreqParam*TC)); ...
        -cos(TimePeriod*tanh(FreqParam*TC)); TimePeriod*tanh(FreqParam*TC)];
    xd31=[-0.5;-0.5;0];
    xd21=[0.5;-0.5;0];
    xd23=xd21-xd31;
    XC=[EC(1:3,:)+X0C;...
        (1/2)*(2*EC(1:3,:)+EC(4:6,:)+EC(7:9,:)+xd21+xd31+xd23+2*X0C);...
        EC(1:3,:)+EC(7:9,:)+xd31+X0C;...
        ];
    N = size(XC,2); %Number of points
else
    N=1;
    NN=1;
    EC=unifrnd(-s2,s2,3*n,N);
    TC=unifrnd(0,1*TimePeriod,1,NN);
    X0C=[sin(TimePeriod*tanh(FreqParam*TC)); ...
    -cos(TimePeriod*tanh(FreqParam*TC)); TimePeriod*tanh(FreqParam*TC)];
    XC=[EC(1:3,:)+X0C;...
        (1/2)*(2*EC(1:3,:)+EC(4:6,:)+EC(7:9,:)+xd21+xd31+xd23+2*X0C);...
        EC(1:3,:)+EC(7:9,:)+xd31+X0C;...
        ];
end
clWc2=zeros(size(Wc2H));
clWa2=zeros(size(Wa2H));
CLmatrix2=zeros(size(Wc2H,1),size(Wc2H,1));
CLGamma2=zeros(size(Gamma2));
parfor i=1:N
    e1i=EC(1:n,i);
    x1i=XC(1:n,i);
    e2i=EC(4:6,i);
    x2i=XC(4:6,i);
    e3i=EC(7:9,i);
    x3i=XC(7:9,i);
    calE2i=[e2i;e1i;e3i;x2i];
    calE1i=[e1i;x1i];
    calE3i=[e3i;e1i;x3i];
    [ mu1i,scrG1i,scrF1i,~,~,~ ] = gen1( calE1i,Wa1H,R1 );
    [ mu3i,scrG3i,scrF3i,~,~,~ ] = gen3( calE3i,calE1i,Wa3H,R2 );
    [ mu2i,scrG2i,scrF2i,calG2i,calF2i,Gsig2i,~ ] = gen2( calE2i,calE1i,calE3i,Wa2H,R2 );
    [~,sig2GRe2i,sig2GRx2i,sig2GRe1i,sig2GRe3i,~]=ADPSEMREMKNN_Basis2(calE2i);
    muS2i=[mu2i;mu1i;mu3i];
    muS3i=[mu3i;mu1i];
    muS1i=mu1i;
    omega2i = sig2GRe2i*(scrF2i+scrG2i*muS2i)+sig2GRx2i*(calF2i+calG2i*muS2i)...
        +sig2GRe1i*(scrF1i+scrG1i*muS1i)+sig2GRe3i*(scrF3i+scrG3i*muS3i);
    ri = e2i'*Q2*e2i + mu2i'*R2*mu2i;
    delta2i = Wc2H'*omega2i + ri;
    rho2i = (1+v2*(omega2i'*omega2i));
    clWc2=clWc2+Gamma2*omega2i*delta2i/rho2i;
    clWa2=clWa2+(Gsig2i'*(R2\Gsig2i))*Wa2H*omega2i'*Wc2H/(4*rho2i);
    CLmatrix2=CLmatrix2+omega2i*omega2i'/(N*rho2i);
    CLGamma2=CLGamma2+Gamma2*(omega2i*omega2i'/rho2i^2)*Gamma2;
end
clWc2=-etac22*clWc2/N;
clWa2=etac22*clWa2/N;
CLGamma2=CLGamma2/N;
cbar2=real(min(svd(CLmatrix2)));

%% Update Laws

Wc2HD = (-etac12*Gamma2*omega2*delta2/rho2+clWc2);
Gamma2D = (beta2*Gamma2-Gamma2*(omega2*omega2'/rho2^2)*Gamma2-CLGamma2);
Wa2HD = etaa12*(Wc2H-Wa2H)...
    -(etaa22*Wa2H-etac12*(Gsig2'*(R2\Gsig2))*Wa2H*omega2'*Wc2H/(4*rho2))+clWa2;
%% Controller
u2 = scrLg22*(muS2+F2);
% u1 = -100*g1'*e1+u10;

== matlab function ADPSEMREMKNNash2015b/Follower 2/Plant/Plant ==
  data: xD output; x input; mu input
function xD = dynamics(x,mu)
%#codegen
F=0;
G=[cos(x(3)) 0;sin(x(3)) 0;0 1];
xD = F+G*mu;

% G=[1 0;0 1;-x(2) x(1)];
% 
% % gplus=
% (1/(x1^2 + x2^2 + 1))*[...
% [ (x1^2 + 1),    (x1*x2), -x2]
% [    (x1*x2), (x2^2 + 1),  x1]];

== matlab function ADPSEMREMKNNash2015b/Follower 4/ADP ==
  data: Wc4H input; Wa4H input; Gamma4 input; x4 input; x0 input; x5 input; e5 input; Wa5H input; t input; R4 parameter; R5 parameter; Q4 parameter; etaa14 parameter; Wc4HD output; Wa4HD output; Gamma4D output; u4 output; clWc4 output; cbar4 output; etaa24 parameter; etac14 parameter; v4 parameter; etac24 parameter; beta4 parameter; n parameter; s4 parameter; MovePoints parameter; xd54 parameter; xd40 parameter; xd45 parameter; e4 output
function [Wc4HD,Wa4HD,Gamma4D,u4,clWc4,cbar4,e4]=...
    control(Wc4H,Wa4H,Gamma4,x4,x0,x5,e5,Wa5H,t,R4,R5,Q4,etaa14,etaa24,etac14,v4,...
    etac24,beta4,n,s4,MovePoints,xd54,xd40,xd45)
%#codegen
e4 = x4-x0-xd40+x4-x5-xd45;
% Z = [e1;x0];
calE4=[e4;e5;x4];
calE5=[e5;e4;x5];
%% ADP
[ mu5,scrG5,scrF5,~,~,~,~ ] = gen5( calE5,calE4,Wa5H,R5,xd40,xd45  );
[ mu4,scrG4,scrF4,calG4,calF4,Gsig4,~,~ ] = gen4( calE4,calE5,Wa4H,R4,xd40,xd45  );
[~,sig4GRe4,sig4GRx4,sig4GRe5,~]=ADPSEMREMKNN_Basis4(calE4); 
muS4=[mu4;mu5];
muS5=[mu5;mu4];
omega4 = sig4GRe4*(scrF4+scrG4*muS4)+sig4GRx4*(calF4+calG4*muS4)...
    +sig4GRe5*(scrF5+scrG5*muS5);
r = e4'*Q4*e4 + mu4'*R4*mu4;
delta4 = Wc4H'*omega4 + r;
rho4 = (1+v4*(omega4'*omega4));
scrLg44=[eye(2) eye(2)];
%% Concurrent Learning
TimePeriod = 6*pi;
FreqParam = 0.1;
if MovePoints == 0
    temp=linspace(-s4,s4,5);
    ttemp=linspace(0,TimePeriod,10);
    [temp1, temp2, temp4] = ndgrid(temp,temp,temp,ttemp);
    EC=[temp1(:) temp2(:)]'; % matrix with columns as selected points
    TC=temp4(:)';
    X0C=[sin(TimePeriod*tanh(FreqParam*TC)); ...
        -cos(TimePeriod*tanh(FreqParam*TC)); TimePeriod*tanh(FreqParam*TC)];
    XC=[EC(1:3,:)+EC(4:6,:)+X0C+xd40+xd45+xd54;...
        2*EC(4:6,:)+EC(1:3,:)+xd40+xd54+xd45+X0C;...
        ];
    N = size(XC,2); %Number of points
else
    N=1;
    NN=1;
    EC=unifrnd(-s4,s4,2*n,N);
    TC=unifrnd(0,1*TimePeriod,1,NN);
    X0C=[sin(TimePeriod*tanh(FreqParam*TC)); ...
    -cos(TimePeriod*tanh(FreqParam*TC)); TimePeriod*tanh(FreqParam*TC)];
    XC=[EC(1:3,:)+EC(4:6,:)+X0C+xd40+xd45+xd54;...
        2*EC(4:6,:)+EC(1:3,:)+xd40+xd54+xd45+X0C;...
        ];
end
clWc4=zeros(size(Wc4H));
clWa4=zeros(size(Wa4H));
CLmatrix4=zeros(size(Wc4H,1),size(Wc4H,1));
CLGamma4=zeros(size(Gamma4));
parfor i=1:N
    e4i=EC(1:3,i);
    x4i=XC(1:3,i);
    e5i=EC(4:6,i);
    x5i=XC(4:6,i);
    calE4i=[e4i;e5i;x4i];
    calE5i=[e5i;e4i;x5i];
    [ mu5i,scrG5i,scrF5i,~,~,~,~ ] = gen5( calE5i,calE4i,Wa5H,R4,xd40,xd45 );
    [ mu4i,scrG4i,scrF4i,calG4i,calF4i,Gsig4i,~,~ ] = gen4( calE4i,calE5i,Wa4H,R4,xd40,xd45 );
    [~,sig4GRe4i,sig4GRx4i,sig4GRe5i,~]=ADPSEMREMKNN_Basis4(calE4i);
    muS4i=[mu4i;mu5i];
    muS5i=[mu5i;mu4i];
    omega4i = sig4GRe4i*(scrF4i+scrG4i*muS4i)+sig4GRx4i*(calF4i+calG4i*muS4i)...
        +sig4GRe5i*(scrF5i+scrG5i*muS5i);
    ri = e4i'*Q4*e4i + mu4i'*R4*mu4i;
    delta4i = Wc4H'*omega4i + ri;
    rho4i = (1+v4*(omega4i'*omega4i));
    clWc4=clWc4+Gamma4*omega4i*delta4i/rho4i;
    clWa4=clWa4+(Gsig4i'*(R4\Gsig4i))*Wa4H*omega4i'*Wc4H/(4*rho4i);
    CLmatrix4=CLmatrix4+omega4i*omega4i'/(N*rho4i);
    CLGamma4=CLGamma4+Gamma4*(omega4i*omega4i'/rho4i^2)*Gamma4;
end
clWc4=-etac24*clWc4/N;
clWa4=etac24*clWa4/N;
CLGamma4=CLGamma4/N;
cbar4=real(min(svd(CLmatrix4)));

%% Update Laws

Wc4HD = (-etac14*Gamma4*omega4*delta4/rho4+clWc4);
Gamma4D = (beta4*Gamma4-Gamma4*(omega4*omega4'/rho4^2)*Gamma4-CLGamma4);
Wa4HD = etaa14*(Wc4H-Wa4H)...
    -(etaa24*Wa4H-etac14*(Gsig4'*(R4\Gsig4))*Wa4H*omega4'*Wc4H/(4*rho4))+clWa4;
%% Controller
[ f0, f40 ] = gen0( x0 );
f45 = [0;0];
f54 = [0;0];
F4 = [f40+f45;f54];
u4 = scrLg44*(muS4+F4);
% u4 = scrLg44*(F4);

== matlab function ADPSEMREMKNNash2015b/Follower 4/Plant/Plant ==
  data: xD output; x input; mu input
function xD = dynamics(x,mu)
%#codegen
F=0;
G=[cos(x(3)) 0;sin(x(3)) 0;0 1];
xD = F+G*mu;

% G=[1 0;0 1;-x(2) x(1)];
% 
% % gplus=
% (1/(x1^2 + x2^2 + 1))*[...
% [ (x1^2 + 1),    (x1*x2), -x2]
% [    (x1*x2), (x2^2 + 1),  x1]];

== matlab function ADPSEMREMKNNash2015b/Follower 5/ADP ==
  data: Wc5H input; Wa5H input; Gamma5 input; x5 input; x4 input; e4 input; Wa4H input; t input; R5 parameter; R4 parameter; Q5 parameter; etaa15 parameter; etaa25 parameter; Wc5HD output; Wa5HD output; Gamma5D output; u5 output; clWc5 output; cbar5 output; e5 output; etac15 parameter; v5 parameter; etac25 parameter; beta5 parameter; n parameter; s5 parameter; MovePoints parameter; xd45 parameter; xd40 parameter; xd54 parameter
function [Wc5HD,Wa5HD,Gamma5D,u5,clWc5,cbar5,e5]=...
    control(Wc5H,Wa5H,Gamma5,x5,x4,e4,Wa4H,t,R5,R4,Q5,etaa15,etaa25,etac15,v5,...
    etac25,beta5,n,s5,MovePoints,xd45,xd40,xd54)
%#codegen
e5 = x5-x4-xd54;
% Z = [e1;x0];
calE5=[e5;e4;x5];
calE4=[e4;e5;x4];
%% ADP
[ mu4,scrG4,scrF4,~,~,~,~,~ ] = gen4( calE4,calE5,Wa4H,R4,xd40,xd45 );
[ mu5,scrG5,scrF5,calG5,calF5,Gsig5,F5 ] = gen5( calE5,calE4,Wa5H,R5,xd40,xd45 );
[~,sig5GRe5,sig5GRx5,sig5GRe4,~]=ADPSEMREMKNN_Basis5(calE5); 
muS5=[mu5;mu4];
muS4=[mu4;mu5];
omega5 = sig5GRe5*(scrF5+scrG5*muS5)+sig5GRx5*(calF5+calG5*muS5)...
    +sig5GRe4*(scrF4+scrG4*muS4);
r = e5'*Q5*e5 + mu5'*R5*mu5;
delta5 = Wc5H'*omega5 + r;
rho5 = (1+v5*(omega5'*omega5));
scrLg55=[2*eye(2) eye(2)];
%% Concurrent Learning
TimePeriod = 6*pi;
FreqParam = 0.1;
if MovePoints == 0
    temp=linspace(-s5,s5,5);
    ttemp=linspace(0,TimePeriod,10);
    [temp1, temp2, temp5] = ndgrid(temp,temp,temp,ttemp);
    EC=[temp1(:) temp2(:)]'; % matrix with columns as selected points
    TC=temp5(:)';
    X0C=[sin(TimePeriod*tanh(FreqParam*TC)); ...
        -cos(TimePeriod*tanh(FreqParam*TC)); TimePeriod*tanh(FreqParam*TC)];
    XC=[EC(1:3,:)+EC(4:6,:)+X0C+xd40+xd54+xd45;...
        2*EC(4:6,:)+EC(1:3,:)+xd40+xd45+xd54+X0C;...
        ];
    N = size(XC,2); %Number of points
else
    N=1;
    NN=1;
    EC=unifrnd(-s5,s5,2*n,N);
    TC=unifrnd(0,1*TimePeriod,1,NN);
    X0C=[sin(TimePeriod*tanh(FreqParam*TC)); ...
    -cos(TimePeriod*tanh(FreqParam*TC)); TimePeriod*tanh(FreqParam*TC)];
    XC=[EC(1:3,:)+EC(4:6,:)+X0C+xd40+xd54+xd45;...
        2*EC(4:6,:)+EC(1:3,:)+xd40+xd45+xd54+X0C;...
        ];
end
clWc5=zeros(size(Wc5H));
clWa5=zeros(size(Wa5H));
CLmatrix5=zeros(size(Wc5H,1),size(Wc5H,1));
CLGamma5=zeros(size(Gamma5));
parfor i=1:N
    e5i=EC(1:3,i);
    x5i=XC(1:3,i);
    e4i=EC(4:6,i);
    x4i=XC(4:6,i);
    calE5i=[e5i;e4i;x5i];
    calE4i=[e4i;e5i;x4i];
    [ mu4i,scrG4i,scrF4i,~,~,~,~,~ ] = gen4( calE4i,calE5i,Wa4H,R5,xd40,xd45  );
    [ mu5i,scrG5i,scrF5i,calG5i,calF5i,Gsig5i,~ ] = gen5( calE5i,calE4i,Wa5H,R5,xd40,xd45  );
    [~,sig5GRe5i,sig5GRx5i,sig5GRe4i,~]=ADPSEMREMKNN_Basis5(calE5i);
    muS5i=[mu5i;mu4i];
    muS4i=[mu4i;mu5i];
    omega5i = sig5GRe5i*(scrF5i+scrG5i*muS5i)+sig5GRx5i*(calF5i+calG5i*muS5i)...
        +sig5GRe4i*(scrF4i+scrG4i*muS4i);
    ri = e5i'*Q5*e5i + mu5i'*R5*mu5i;
    delta5i = Wc5H'*omega5i + ri;
    rho5i = (1+v5*(omega5i'*omega5i));
    clWc5=clWc5+Gamma5*omega5i*delta5i/rho5i;
    clWa5=clWa5+(Gsig5i'*(R5\Gsig5i))*Wa5H*omega5i'*Wc5H/(4*rho5i);
    CLmatrix5=CLmatrix5+omega5i*omega5i'/(N*rho5i);
    CLGamma5=CLGamma5+Gamma5*(omega5i*omega5i'/rho5i^2)*Gamma5;
end
clWc5=-etac25*clWc5/N;
clWa5=etac25*clWa5/N;
CLGamma5=CLGamma5/N;
cbar5=real(min(svd(CLmatrix5)));

%% Update Laws

Wc5HD = (-etac15*Gamma5*omega5*delta5/rho5+clWc5);
Gamma5D = (beta5*Gamma5-Gamma5*(omega5*omega5'/rho5^2)*Gamma5-CLGamma5);
Wa5HD = etaa15*(Wc5H-Wa5H)...
    -(etaa25*Wa5H-etac15*(Gsig5'*(R5\Gsig5))*Wa5H*omega5'*Wc5H/(4*rho5))+clWa5;
%% Controller
u5 = scrLg55*(muS5+F5);
% u5 = scrLg55*(F5);

== matlab function ADPSEMREMKNNash2015b/Follower 5/Plant/Plant ==
  data: xD output; x input; mu input
function xD = dynamics(x,mu)
%#codegen
F=0;
G=[cos(x(3)) 0;sin(x(3)) 0;0 1];
xD = F+G*mu;

% G=[1 0;0 1;-x(2) x(1)];
% 
% % gplus=
% (1/(x1^2 + x2^2 + 1))*[...
% [ (x1^2 + 1),    (x1*x2), -x2]
% [    (x1*x2), (x2^2 + 1),  x1]];
